simulink model "gastrointestinal"  (R2023a)
settings: Solver=ode23t  StartTime=0.0  StopTime=10  MaxStep=1E-3  RelTol=1e-3
libraries: fl_lib x18, nesl_utility x6, slpidlib x1
settings Model: LastModifiedBy=santi
settings DataIOCC: ReturnWorkspaceOutputs=off  TimeSaveName=t
settings DebuggingCC: AlgebraicLoopMsg=none  ArtificialAlgebraicLoopMsg=none  MaxConsecutiveZCsMsg=none
settings RTWCC: GPUComputeCapability=5.0

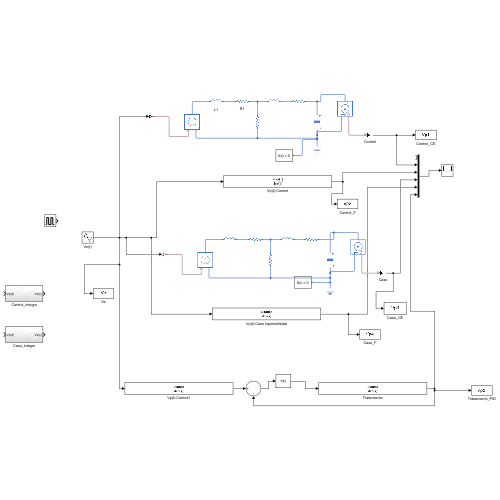
[thumbnail: Simulink's stored preview of the top-level diagram]
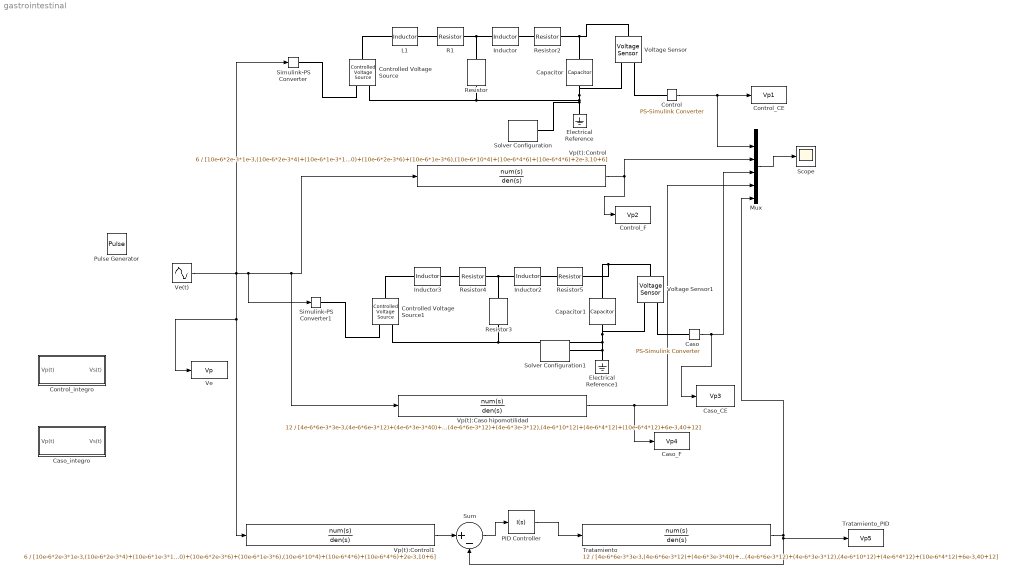
== system gastrointestinal ==
  Capacitor : fl_lib/Electrical/Electrical Elements/Capacitor  c=10e-6 F  r=0 Ohm  g=0 1/Ohm  i_specify=off  i_priority=None  i=0 A  i_nominal_specify=off  i_nominal_unit=A  i_nominal_value=1  v_specify=off  v_priority=None  v=0 V  v_nominal_specify=off  v_nominal_unit=V  v_nominal_value=1  vc_specify=off  vc_priority=High  vc=0 V  vc_nominal_specify=off  vc_nominal_unit=V  vc_nominal_value=1
  Capacitor1 : fl_lib/Electrical/Electrical Elements/Capacitor  c=4e-6 F  r=0 Ohm  g=0 1/Ohm  i_specify=off  i_priority=None  i=0 A  i_nominal_specify=off  i_nominal_unit=A  i_nominal_value=1  v_specify=off  v_priority=None  v=0 V  v_nominal_specify=off  v_nominal_unit=V  v_nominal_value=1  vc_specify=off  vc_priority=High  vc=0 V  vc_nominal_specify=off  vc_nominal_unit=V  vc_nominal_value=1
  Caso : nesl_utility/PS-Simulink Converter  PhysicalDomain=network_engine_domain  SubClassName=ps_output  LeftPortType=input  RightPortType=output  PseudoPeriodic=off  Frequencies=[]  VectorFormat=1-D array  Unit=inherit  AffineConversion=off
  Caso_CE : ToWorkspace  VariableName=Vp3  SampleTime=-1
      settings: Save2DSignal=2-D array (concatenate along first dimension)
  Caso_F : ToWorkspace  VariableName=Vp4  SampleTime=-1
      settings: Save2DSignal=2-D array (concatenate along first dimension)
  Caso_integro : Subsystem
  Control : nesl_utility/PS-Simulink Converter  PhysicalDomain=network_engine_domain  SubClassName=ps_output  LeftPortType=input  RightPortType=output  PseudoPeriodic=off  Frequencies=[]  VectorFormat=1-D array  Unit=inherit  AffineConversion=off
  Control_CE : ToWorkspace  VariableName=Vp1  SampleTime=-1
      settings: Save2DSignal=2-D array (concatenate along first dimension)
  Control_F : ToWorkspace  VariableName=Vp2  SampleTime=-1
      settings: Save2DSignal=2-D array (concatenate along first dimension)
  Control_integro : Subsystem
  Controlled Voltage Source : fl_lib/Electrical/Electrical Sources/Controlled Voltage Source
  Controlled Voltage Source1 : fl_lib/Electrical/Electrical Sources/Controlled Voltage Source
  Electrical Reference : fl_lib/Electrical/Electrical Elements/Electrical Reference
  Electrical Reference1 : fl_lib/Electrical/Electrical Elements/Electrical Reference
  Inductor : fl_lib/Electrical/Electrical Elements/Inductor  l=1e-3 H  r=0 Ohm  g=1e-9 1/Ohm  i_specify=off  i_priority=None  i=0 A  i_nominal_specify=off  i_nominal_unit=A  i_nominal_value=1  v_specify=off  v_priority=None  v=0 V  v_nominal_specify=off  v_nominal_unit=V  v_nominal_value=1  i_L_specify=off  i_L_priority=High  i_L=0 A  i_L_nominal_specify=off  i_L_nominal_unit=A  i_L_nominal_value=1
  Inductor2 : fl_lib/Electrical/Electrical Elements/Inductor  l=3e-3 H  r=0 Ohm  g=1e-9 1/Ohm  i_specify=off  i_priority=None  i=0 A  i_nominal_specify=off  i_nominal_unit=A  i_nominal_value=1  v_specify=off  v_priority=None  v=0 V  v_nominal_specify=off  v_nominal_unit=V  v_nominal_value=1  i_L_specify=off  i_L_priority=High  i_L=0 A  i_L_nominal_specify=off  i_L_nominal_unit=A  i_L_nominal_value=1
  Inductor3 : fl_lib/Electrical/Electrical Elements/Inductor  l=6e-3 H  r=0 Ohm  g=1e-9 1/Ohm  i_specify=off  i_priority=None  i=0 A  i_nominal_specify=off  i_nominal_unit=A  i_nominal_value=1  v_specify=off  v_priority=None  v=0 V  v_nominal_specify=off  v_nominal_unit=V  v_nominal_value=1  i_L_specify=off  i_L_priority=High  i_L=0 A  i_L_nominal_specify=off  i_L_nominal_unit=A  i_L_nominal_value=1
  L1 : fl_lib/Electrical/Electrical Elements/Inductor  l=2e-3 H  r=0 Ohm  g=1e-9 1/Ohm  i_specify=off  i_priority=None  i=0 A  i_nominal_specify=off  i_nominal_unit=A  i_nominal_value=1  v_specify=off  v_priority=None  v=0 V  v_nominal_specify=off  v_nominal_unit=V  v_nominal_value=1  i_L_specify=off  i_L_priority=High  i_L=0 A  i_L_nominal_specify=off  i_L_nominal_unit=A  i_L_nominal_value=1
  Mux : Mux  Inputs=6
  PID Controller : slpidlib/PID Controller  Controller=I  Form=Parallel  TimeDomain=Continuous-time  UseExternalTs=off  SampleTime=-1  IntegratorMethod=Forward Euler  FilterMethod=Forward Euler  ControllerParametersSource=internal  P=0  I=7139.66929170782  UseKiTs=off  D=0  N=100  UseFilter=on  TunerSelectOption=Transfer Function Based (PID Tuner App)  InitialConditionSource=internal  InitialConditionForIntegrator=0  InitialConditionForFilter=0  DifferentiatorICPrevScaledInput=0  ExternalReset=none  TrackingMode=off  Kt=1  LimitOutput=off  SatLimitsSource=internal  UpperSaturationLimit=inf  LowerSaturationLimit=-inf  LinearizeAsGain=on  AntiWindupMode=none  Kb=1  LimitIntegrator=off  UpperIntegratorSaturationLimit=inf  LowerIntegratorSaturationLimit=-inf  POutMin=[]  POutMax=[]  IOutMin=[]  IOutMax=[]  DOutMin=[]  DOutMax=[]  NOutMin=[]  NOutMax=[]  SumOutMin=[]  SumOutMax=[]  SaturationOutMin=[]  SaturationOutMax=[]  PParamMin=[]  PParamMax=[]  IParamMin=[]  IParamMax=[]  DParamMin=[]  DParamMax=[]  NParamMin=[]  NParamMax=[]  KbParamMin=[]  KbParamMax=[]  KtParamMin=[]  KtParamMax=[]  KbOutMin=[]  KbOutMax=[]  KtOutMin=[]  KtOutMax=[]  IntegratorOutMin=[]  IntegratorOutMax=[]  FilterOutMin=[]  FilterOutMax=[]  SumI1OutMin=[]  SumI1OutMax=[]  SumI2OutMin=[]  SumI2OutMax=[]  SumI3OutMin=[]  SumI3OutMax=[]  SumI4OutMin=[]  SumI4OutMax=[]  SumDOutMin=[]  SumDOutMax=[]  DifferentiatorOutMin=[]  DifferentiatorOutMax=[]  FilterDiffOutCoefMin=[]  FilterDiffOutCoefMax=[]  ReciprocalOutMin=[]  ReciprocalOutMax=[]  SumDenOutMin=[]  SumDenOutMax=[]  SumNumOutMin=[]  SumNumOutMax=[]  DivideOutMin=[]  DivideOutMax=[]  UdiffTsProdOutMin=[]  UdiffTsProdOutMax=[]  NTsProdOutMin=[]  NTsProdOutMax=[]  UintegralTsProdOutMin=[]  UintegralTsProdOutMax=[]  UngainTsProdOutMin=[]  UngainTsProdOutMax=[]  ClampingZeroOutDataTypeStr=Inherit: Inherit via back propagation  ClampingZeroOutMin=[]  ClampingZeroOutMax=[]  FilterDenConstantOutDataTypeStr=Inherit: Inherit via back propagation  FilterDenConstantOutMin=[]  FilterDenConstantOutMax=[]  PCopyOutDataTypeStr=Inherit: Inherit via back propagation  PCopyOutMin=[]  PCopyOutMax=[]  NCopyOutDataTypeStr=Inherit: Inherit via back propagation  NCopyOutMin=[]  NCopyOutMax=[]  IntegratorContinuousStateAttributes=''  IntegratorStateMustResolveToSignalObject=off  IntegratorRTWStateStorageClass=Auto  FilterContinuousStateAttributes=''  FilterStateMustResolveToSignalObject=off  FilterRTWStateStorageClass=Auto  ParallelPVariant=Disabled  IdealPVariant=Disabled  IVariant=InternalParameters  DVariant=Disabled  IntegratorVariant=Continuous  SatVariant=Disabled  AWVariant=Passthrough  PCopyVariant=Disabled  TRVariant=Disabled  FdbkBlocksVariant=Forward  IdealPFdbkVariant=Disabled  SatFdbkVariant=Disabled  DerivativeFilterVariant=Disabled  NVariant=Disabled  NCopyVariant=Disabled_SignalSpec  FilterICVariant=Disabled  IntegratorICVariant=InternalICs  ExternalResetVariant=Disabled  TRSumVariant=Passthrough  SumFdbkVariant=Disabled  SumVariant=Passthrough_I  TsampFilterVariant=InternalTs  TsampNgainVariant=Passthrough  TsampIntegralVariant=Disabled_SignalSpec  ExternalSaturationOutDataTypeStr=Inherit: Same as second input
  Pulse Generator : DiscretePulseGenerator  PulseType=Time based  Period=10  PulseWidth=5
  R1 : fl_lib/Electrical/Electrical Elements/Resistor  R=10 Ohm  i_specify=off  i_priority=None  i=0 A  i_nominal_specify=off  i_nominal_unit=A  i_nominal_value=1  v_specify=off  v_priority=None  v=0 V  v_nominal_specify=off  v_nominal_unit=V  v_nominal_value=1
  Resistor : fl_lib/Electrical/Electrical Elements/Resistor  R=6 Ohm  i_specify=off  i_priority=None  i=0 A  i_nominal_specify=off  i_nominal_unit=A  i_nominal_value=1  v_specify=off  v_priority=None  v=0 V  v_nominal_specify=off  v_nominal_unit=V  v_nominal_value=1
  Resistor2 : fl_lib/Electrical/Electrical Elements/Resistor  R=4 Ohm  i_specify=off  i_priority=None  i=0 A  i_nominal_specify=off  i_nominal_unit=A  i_nominal_value=1  v_specify=off  v_priority=None  v=0 V  v_nominal_specify=off  v_nominal_unit=V  v_nominal_value=1
  Resistor3 : fl_lib/Electrical/Electrical Elements/Resistor  R=12 Ohm  i_specify=off  i_priority=None  i=0 A  i_nominal_specify=off  i_nominal_unit=A  i_nominal_value=1  v_specify=off  v_priority=None  v=0 V  v_nominal_specify=off  v_nominal_unit=V  v_nominal_value=1
  Resistor4 : fl_lib/Electrical/Electrical Elements/Resistor  R=40 Ohm  i_specify=off  i_priority=None  i=0 A  i_nominal_specify=off  i_nominal_unit=A  i_nominal_value=1  v_specify=off  v_priority=None  v=0 V  v_nominal_specify=off  v_nominal_unit=V  v_nominal_value=1
  Resistor5 : fl_lib/Electrical/Electrical Elements/Resistor  R=12 Ohm  i_specify=off  i_priority=None  i=0 A  i_nominal_specify=off  i_nominal_unit=A  i_nominal_value=1  v_specify=off  v_priority=None  v=0 V  v_nominal_specify=off  v_nominal_unit=V  v_nominal_value=1
  Scope : Scope
  Simulink-PS Converter : nesl_utility/Simulink-PS Converter  PhysicalDomain=network_engine_domain  SubClassName=ps_input  LeftPortType=input  RightPortType=output  PseudoPeriodic=off  Frequencies=[]  NoiseDistribution=none  NoiseParameters=[]  Unit=1  AffineConversion=off  FilteringAndDerivatives=provide  SimscapeFilterOrder=1  InputFilterTimeConstant=0.001  UdotUserProvided=0
  Simulink-PS Converter1 : nesl_utility/Simulink-PS Converter  PhysicalDomain=network_engine_domain  SubClassName=ps_input  LeftPortType=input  RightPortType=output  PseudoPeriodic=off  Frequencies=[]  NoiseDistribution=none  NoiseParameters=[]  Unit=1  AffineConversion=off  FilteringAndDerivatives=provide  SimscapeFilterOrder=1  InputFilterTimeConstant=0.001  UdotUserProvided=0
  Solver Configuration : nesl_utility/Solver Configuration  PhysicalDomain=network_engine_domain  SubClassName=solver  LeftPortType=input  RightPortType=generic  Tones=[]  Harmonics=[]  SimulateNoise=off  Profile=off  UseLocalSampling=off  EnableSwitchedLinearOptims=on  FrequencyDomain=off  UseCCode=off  RelTol=0.001  AbsTol=0.001  MinStep=1e-09  ToWorkspace=off  RevertToSquareIcSolve=off  NumHomotopyIterations=100  PhasorMode=off  PhasorModeNumHarmonics=1  ConsistencySolver=NEWTON_XTOL_AFTER_FTOL  IndexReductionMethod=DerivativeReplacement  DoDC=off  ResidualTolerance=1e-09  ConsistencyTolSource=GLOBAL  ConsistencyAbsTol=0.001  ConsistencyRelTol=0.001  ConsistencyTolFactor=0.001  UseLocalSolver=off  LocalSolverChoice=NE_BACKWARD_EULER_ADVANCER  ResolveIndetEquations=on  FunctionEvalNumThread=1  LocalSolverSampleTime=0.001  DoFixedCost=off  MaxNonlinIter=3  MaxModeIter=2  ComputeImpulses=off  ImpulseIterations=2  LinearAlgebra=auto  LinearAlgebraNumThread=0  EquationFormulation=NE_TIME_EF  DelaysMemoryBudget=1024  AutomaticFiltering=on  FilteringTimeConstant=0.001  PartitionStorageMethod=AS_NEEDED  PartitionMemoryBudget=1024  PartitionMethod=ROBUST
  Solver Configuration1 : nesl_utility/Solver Configuration  PhysicalDomain=network_engine_domain  SubClassName=solver  LeftPortType=input  RightPortType=generic  Tones=[]  Harmonics=[]  SimulateNoise=off  Profile=off  UseLocalSampling=off  EnableSwitchedLinearOptims=on  FrequencyDomain=off  UseCCode=off  RelTol=0.001  AbsTol=0.001  MinStep=1e-09  ToWorkspace=off  RevertToSquareIcSolve=off  NumHomotopyIterations=100  PhasorMode=off  PhasorModeNumHarmonics=1  ConsistencySolver=NEWTON_XTOL_AFTER_FTOL  IndexReductionMethod=DerivativeReplacement  DoDC=off  ResidualTolerance=1e-09  ConsistencyTolSource=GLOBAL  ConsistencyAbsTol=0.001  ConsistencyRelTol=0.001  ConsistencyTolFactor=0.001  UseLocalSolver=off  LocalSolverChoice=NE_BACKWARD_EULER_ADVANCER  ResolveIndetEquations=on  FunctionEvalNumThread=1  LocalSolverSampleTime=0.001  DoFixedCost=off  MaxNonlinIter=3  MaxModeIter=2  ComputeImpulses=off  ImpulseIterations=2  LinearAlgebra=auto  LinearAlgebraNumThread=0  EquationFormulation=NE_TIME_EF  DelaysMemoryBudget=1024  AutomaticFiltering=on  FilteringTimeConstant=0.001  PartitionStorageMethod=AS_NEEDED  PartitionMemoryBudget=1024  PartitionMethod=ROBUST
  Sum : Sum  Inputs=|+-
  Tratamiento : TransferFcn  Numerator=12  Denominator=[4e-6*6e-3*3e-3,(4e-6*6e-3*12)+(4e-6*3e-3*40)+(4e-6*6e-3*12)+(4e-6*3e-3*12),(4e-6*10*12)+(4e-6*4*12)+(10e-6*4*12)+6e-3,40+12]
  Tratamiento_PID : ToWorkspace  VariableName=Vp5  SampleTime=-1
      settings: Save2DSignal=2-D array (concatenate along first dimension)
  Ve : ToWorkspace  VariableName=Vp  SampleTime=-1
      settings: Save2DSignal=2-D array (concatenate along first dimension)
  Ve(t) : Sin  SampleTime=0
  Voltage Sensor : fl_lib/Electrical/Electrical Sensors/Voltage Sensor
  Voltage Sensor1 : fl_lib/Electrical/Electrical Sensors/Voltage Sensor
  Vp(t):Caso hipomotilidad : TransferFcn  Numerator=12  Denominator=[4e-6*6e-3*3e-3,(4e-6*6e-3*12)+(4e-6*3e-3*40)+(4e-6*6e-3*12)+(4e-6*3e-3*12),(4e-6*10*12)+(4e-6*4*12)+(10e-6*4*12)+6e-3,40+12]
  Vp(t):Control : TransferFcn  Numerator=6  Denominator=[10e-6*2e-3*1e-3,(10e-6*2e-3*4)+(10e-6*1e-3*10)+(10e-6*2e-3*6)+(10e-6*1e-3*6),(10e-6*10*4)+(10e-6*4*6)+(10e-6*4*6)+2e-3,10+6]
  Vp(t):Control1 : TransferFcn  Numerator=6  Denominator=[10e-6*2e-3*1e-3,(10e-6*2e-3*4)+(10e-6*1e-3*10)+(10e-6*2e-3*6)+(10e-6*1e-3*6),(10e-6*10*4)+(10e-6*4*6)+(10e-6*4*6)+2e-3,10+6]
  wires:
  Vp(t):Caso hipomotilidad/1 -> Caso_F/1, Mux/5
  Ve(t)/1 -> Ve/1, Vp(t):Control1/1, Vp(t):Control/1, Vp(t):Caso hipomotilidad/1, Simulink-PS Converter1/1, Simulink-PS Converter/1
  Vp(t):Control/1 -> Mux/3, Control_F/1
  Mux/1 -> Scope/1
  Vp(t):Control1/1 -> Sum/1
  Caso/1 -> Caso_CE/1, Mux/4
  Tratamiento/1 -> Tratamiento_PID/1, Sum/2, Mux/6
  Sum/1 -> PID Controller/1
  PID Controller/1 -> Tratamiento/1
  Control/1 -> Control_CE/1, Mux/2
  connections:
  Capacitor/LConn1 -- Resistor2/RConn1 -- Voltage Sensor/LConn1
  Capacitor1/RConn1 -- Controlled Voltage Source1/RConn2 -- Resistor3/RConn1 -- Solver Configuration1/RConn1 -- Electrical Reference1/LConn1 -- Voltage Sensor1/RConn2
  Resistor3/LConn1 -- Resistor4/RConn1 -- Inductor2/LConn1
  Inductor/LConn1 -- R1/RConn1 -- Resistor/LConn1
  Capacitor1/LConn1 -- Voltage Sensor1/LConn1 -- Resistor5/RConn1
  Resistor/RConn1 -- Capacitor/RConn1 -- Voltage Sensor/RConn2 -- Electrical Reference/LConn1 -- Solver Configuration/RConn1 -- Controlled Voltage Source/RConn2
  L1/RConn1 -- R1/LConn1
  Caso/LConn1 -- Voltage Sensor1/RConn1
  Inductor/RConn1 -- Resistor2/LConn1
  Simulink-PS Converter/RConn1 -- Controlled Voltage Source/RConn1
  Inductor2/RConn1 -- Resistor5/LConn1
  Simulink-PS Converter1/RConn1 -- Controlled Voltage Source1/RConn1
  Control/LConn1 -- Voltage Sensor/RConn1
  L1/LConn1 -- Controlled Voltage Source/LConn1
  Inductor3/LConn1 -- Controlled Voltage Source1/LConn1
  Inductor3/RConn1 -- Resistor4/LConn1

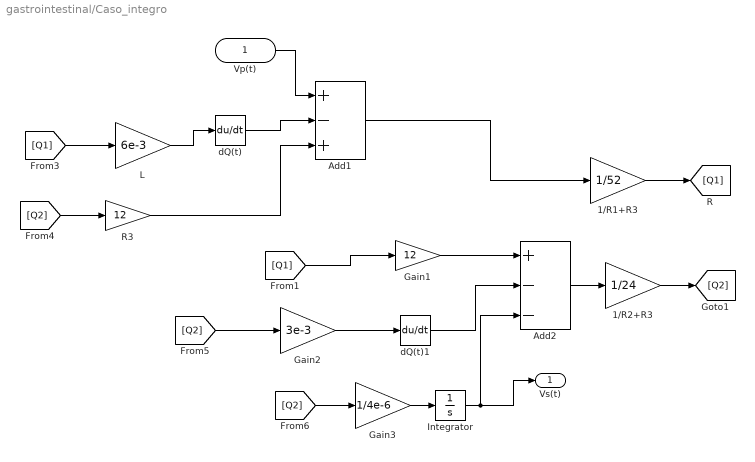
== system gastrointestinal/Caso_integro ==
  Vp(t) : Inport
  1/R1+R3 : Gain  Gain=1/52
  1/R2+R3 : Gain  Gain=1/24
  Add1 : Sum  Inputs=+-+
  Add2 : Sum  Inputs=+--
  Gain1 : Gain  Gain=12
  Gain2 : Gain  Gain=3e-3
  Gain3 : Gain  Gain=1/4e-6
  Integrator : Integrator
  L : Gain  Gain=6e-3
  R3 : Gain  Gain=12
  dQ(t) : Derivative
  dQ(t)1 : Derivative
  Vs(t) : Outport
  wires:
  Add2/1 -> 1/R2+R3/1
  1/R1+R3/1 -> [Q1]
  1/R2+R3/1 -> [Q2]
  Gain3/1 -> Integrator/1
  Gain2/1 -> dQ(t)1/1
  Add1/1 -> 1/R1+R3/1
  Vp(t)/1 -> Add1/1
  Integrator/1 -> Add2/3, Vs(t)/1
  [Q2] -> Gain3/1
  [Q2] -> Gain2/1
  [Q1] -> Gain1/1
  [Q2] -> R3/1
  [Q1] -> L/1
  L/1 -> dQ(t)/1
  dQ(t)/1 -> Add1/2
  R3/1 -> Add1/3
  Gain1/1 -> Add2/1
  dQ(t)1/1 -> Add2/2

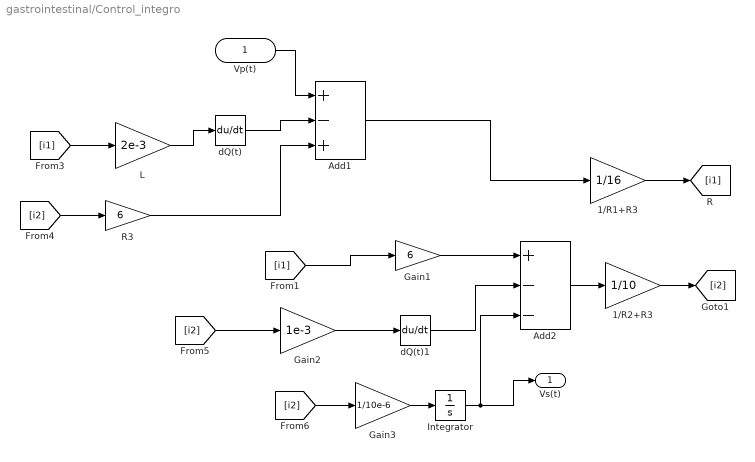
== system gastrointestinal/Control_integro ==
  Vp(t) : Inport
  1/R1+R3 : Gain  Gain=1/16
  1/R2+R3 : Gain  Gain=1/10
  Add1 : Sum  Inputs=+-+
  Add2 : Sum  Inputs=+--
  Gain1 : Gain  Gain=6
  Gain2 : Gain  Gain=1e-3
  Gain3 : Gain  Gain=1/10e-6
  Integrator : Integrator
  L : Gain  Gain=2e-3
  R3 : Gain  Gain=6
  dQ(t) : Derivative
  dQ(t)1 : Derivative
  Vs(t) : Outport
  wires:
  Add2/1 -> 1/R2+R3/1
  1/R1+R3/1 -> [i1]
  1/R2+R3/1 -> [i2]
  Gain3/1 -> Integrator/1
  Gain2/1 -> dQ(t)1/1
  Add1/1 -> 1/R1+R3/1
  Vp(t)/1 -> Add1/1
  Integrator/1 -> Add2/3, Vs(t)/1
  [i2] -> Gain3/1
  [i2] -> Gain2/1
  [i1] -> Gain1/1
  [i2] -> R3/1
  [i1] -> L/1
  L/1 -> dQ(t)/1
  dQ(t)/1 -> Add1/2
  R3/1 -> Add1/3
  Gain1/1 -> Add2/1
  dQ(t)1/1 -> Add2/2
